simulink model "simulink_3K04"  (R2022a)
settings: Solver=FixedStepAuto  StartTime=0.0  StopTime=10.0  FixedStep=1e-3  RelTol=1e-3  EnableMultiTasking=on
undefined symbols (not defined in the file): D0, D1, D10, D11, D12, D13, D2, D3, D4, D5, D6, D7, D8, D9, PTA0, PTA1, PTA2, PTB23, PTB9, PTC16, PTC17, PTC2, PTC3, PTC4, PTD0, PTD1, PTD2, PTD3
libraries: frdmk64flib x19
settings Model: ExtModeTrigDuration=5  Creator=patri  LastModifiedBy=patri
settings OptimizationCC: EnhancedBackFolding=on  PassReuseOutputArgsAs=Individual arguments  ZeroExternalMemoryAtStartup=off  ZeroInternalMemoryAtStartup=off  MaxStackSize=64  OptimizeBlockOrder=speed  DifferentSizesBufferReuse=on  OptimizationCustomize=off  EfficientTunableParamExpr=on
settings DebuggingCC: ParameterTunabilityLossMsg=error
settings HardwareCC: ProdBitPerPointer=32  ProdBitPerSizeT=32  ProdBitPerPtrDiffT=32  ProdLargestAtomicInteger=Long  ProdLargestAtomicFloat=Double  ProdWordSize=32  ProdHWDeviceType=ARM Compatible->ARM Cortex
settings SFSimCC: MATLABDynamicMemAlloc=off
settings RTWCC: SystemTargetFile=ert.tlc  HardwareBoard=NXP FRDM-K64F  TLCOptions="-aInlineSetEventsForThisBaseRateFcn=TLC_FALSE -aSuppressMultiTaskScheduler=TLC_FALSE  -aRateBasedStepFcn=0"  TemplateMakefile=ert_default_tmf  Toolchain=GNU Tools for ARM Embedded Processors
settings CodeAppCC: ForceParamTrailComments=on  IgnoreCustomStorageClasses=off  OperatorAnnotations=on  SimulinkDataObjDesc=on  SFDataObjDesc=on  InsertBlockDesc=on
settings ERTTargetCC: ExtModeTransport=4  ExtModeMexFile=sendToCommService

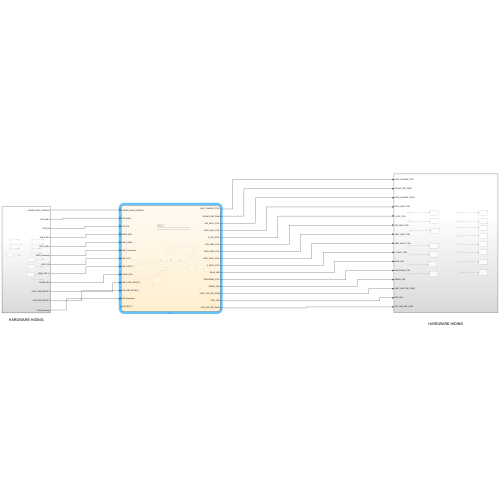
[thumbnail: Simulink's stored preview of the top-level diagram]
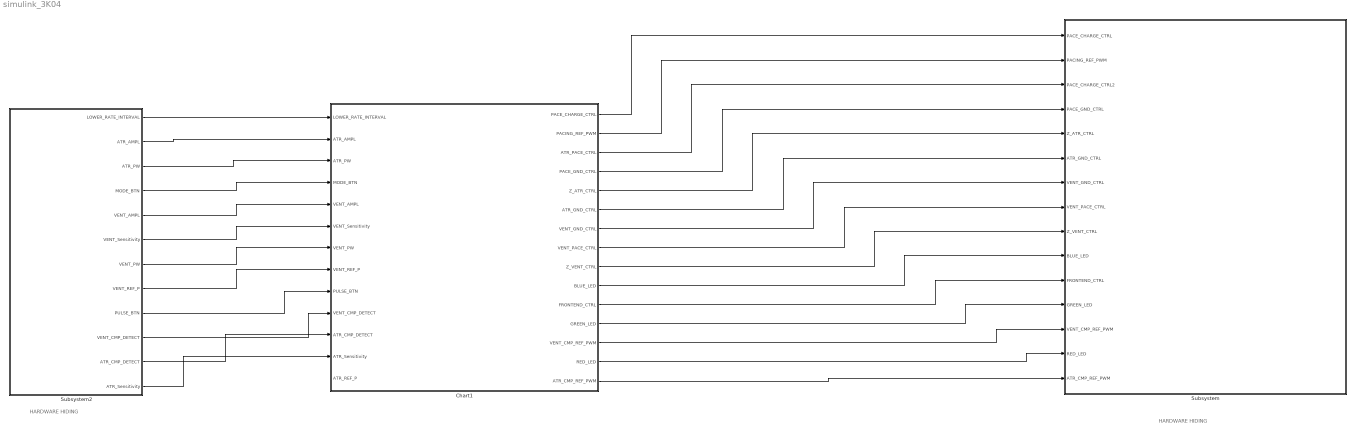
== system simulink_3K04 ==
  note: HARDWARE HIDING
  note: HARDWARE HIDING
  Chart1 : Stateflow chart  TreatAsAtomicUnit=on
  Subsystem : Subsystem
  Subsystem2 : Subsystem
  wires:
  Subsystem2/1(LOWER_RATE_INTERVAL) -> Chart1/1(LOWER_RATE_INTERVAL)
  Chart1/3(ATR_PACE_CTRL) -> Subsystem/3(PACE_CHARGE_CTRL2)
  Chart1/2(PACING_REF_PWM) -> Subsystem/2(PACING_REF_PWM)
  Subsystem2/5(VENT_AMPL) -> Chart1/5(VENT_AMPL)
  Chart1/1(PACE_CHARGE_CTRL) -> Subsystem/1(PACE_CHARGE_CTRL)
  Subsystem2/2(ATR_AMPL) -> Chart1/2(ATR_AMPL)
  Subsystem2/8(VENT_REF_P) -> Chart1/8(VENT_REF_P)
  Chart1/4(PACE_GND_CTRL) -> Subsystem/4(PACE_GND_CTRL)
  Subsystem2/7(VENT_PW) -> Chart1/7(VENT_PW)
  Subsystem2/4(MODE_BTN) -> Chart1/4(MODE_BTN)
  Chart1/7(VENT_GND_CTRL) -> Subsystem/7(VENT_GND_CTRL)
  Chart1/8(VENT_PACE_CTRL) -> Subsystem/8(VENT_PACE_CTRL)
  Chart1/6(ATR_GND_CTRL) -> Subsystem/6(ATR_GND_CTRL)
  Subsystem2/6(VENT_Sensitivity) -> Chart1/6(VENT_Sensitivity)
  Subsystem2/3(ATR_PW) -> Chart1/3(ATR_PW)
  Subsystem2/9(PULSE_BTN) -> Chart1/9(PULSE_BTN)
  Subsystem2/10(VENT_CMP_DETECT) -> Chart1/10(VENT_CMP_DETECT)
  Chart1/11(FRONTEND_CTRL) -> Subsystem/11(FRONTEND_CTRL)
  Chart1/14(RED_LED) -> Subsystem/14(RED_LED)
  Chart1/9(Z_VENT_CTRL) -> Subsystem/9(Z_VENT_CTRL)
  Chart1/12(GREEN_LED) -> Subsystem/12(GREEN_LED)
  Chart1/5(Z_ATR_CTRL) -> Subsystem/5(Z_ATR_CTRL)
  Chart1/13(VENT_CMP_REF_PWM) -> Subsystem/13(VENT_CMP_REF_PWM)
  Chart1/10(BLUE_LED) -> Subsystem/10(BLUE_LED)
  Subsystem2/11(ATR_CMP_DETECT) -> Chart1/11(ATR_CMP_DETECT)
  Chart1/15(ATR_CMP_REF_PWM) -> Subsystem/15(ATR_CMP_REF_PWM)
  Subsystem2/12(ATR_Sensitivity) -> Chart1/12(ATR_Sensitivity)

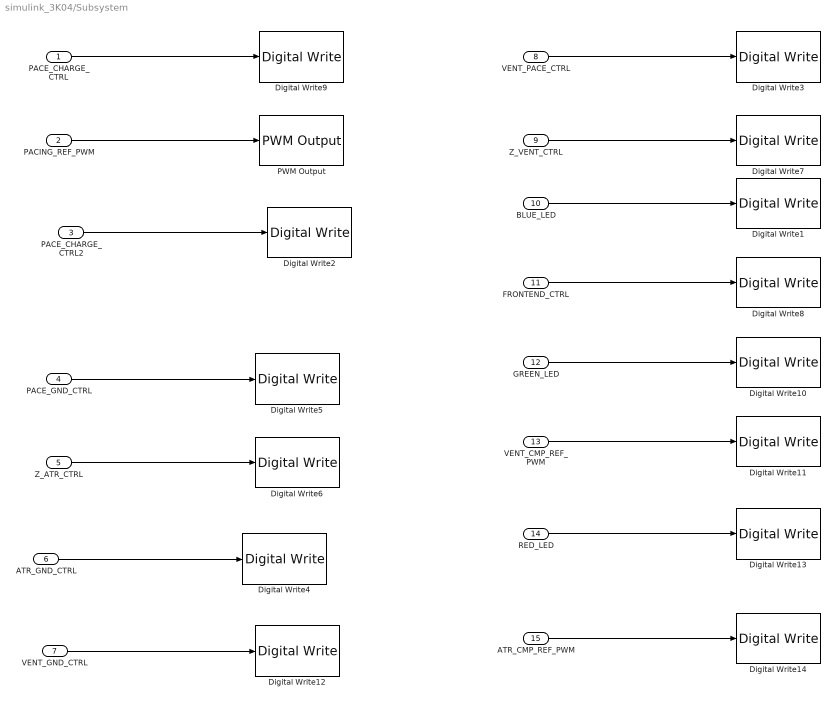
== system simulink_3K04/Subsystem ==
  PACE_CHARGE_CTRL : Inport
  PACING_REF_PWM : Inport  Port=2
  PACE_CHARGE_CTRL2 : Inport  Port=3
  PACE_GND_CTRL : Inport  Port=4
  Z_ATR_CTRL : Inport  Port=5
  ATR_GND_CTRL : Inport  Port=6
  VENT_GND_CTRL : Inport  Port=7
  VENT_PACE_CTRL : Inport  Port=8
  Z_VENT_CTRL : Inport  Port=9
  BLUE_LED : Inport  Port=10
  FRONTEND_CTRL : Inport  Port=11
  GREEN_LED : Inport  Port=12
  VENT_CMP_REF_PWM : Inport  Port=13
  RED_LED : Inport  Port=14
  ATR_CMP_REF_PWM : Inport  Port=15
  Digital Write1 : frdmk64flib/Digital Write  Whichpin=BLUE_LED
  Digital Write10 : frdmk64flib/Digital Write  Whichpin=GREEN_LED
  Digital Write11 : frdmk64flib/Digital Write  Whichpin=PTA1 (D3)
  Digital Write12 : frdmk64flib/Digital Write  Whichpin=PTD3 (D12)
  Digital Write13 : frdmk64flib/Digital Write  Whichpin=RED_LED
  Digital Write14 : frdmk64flib/Digital Write  Whichpin=PTC2 (D6)
  Digital Write2 : frdmk64flib/Digital Write  Whichpin=PTA0 (D8)
  Digital Write3 : frdmk64flib/Digital Write  Whichpin=PTC4 (D9)
  Digital Write4 : frdmk64flib/Digital Write  Whichpin=PTD2 (D11)
  Digital Write5 : frdmk64flib/Digital Write  Whichpin=PTD0 (D10)
  Digital Write6 : frdmk64flib/Digital Write  Whichpin=PTB23 (D4)
  Digital Write7 : frdmk64flib/Digital Write  Whichpin=PTC3 (D7)
  Digital Write8 : frdmk64flib/Digital Write  Whichpin=PTD1 (D13)
  Digital Write9 : frdmk64flib/Digital Write  Whichpin=PTB9 (D2)
  PWM Output : frdmk64flib/PWM Output  Whichpin=PTA2 (D5)  InitialFrequency=2000  InitialDutyCycle=0
  wires:
  PACE_CHARGE_CTRL/1 -> Digital Write9/1
  PACING_REF_PWM/1 -> PWM Output/1
  PACE_CHARGE_CTRL2/1 -> Digital Write2/1
  PACE_GND_CTRL/1 -> Digital Write5/1
  Z_ATR_CTRL/1 -> Digital Write6/1
  ATR_GND_CTRL/1 -> Digital Write4/1
  VENT_GND_CTRL/1 -> Digital Write12/1
  VENT_PACE_CTRL/1 -> Digital Write3/1
  Z_VENT_CTRL/1 -> Digital Write7/1
  BLUE_LED/1 -> Digital Write1/1
  FRONTEND_CTRL/1 -> Digital Write8/1
  GREEN_LED/1 -> Digital Write10/1
  VENT_CMP_REF_PWM/1 -> Digital Write11/1
  RED_LED/1 -> Digital Write13/1
  ATR_CMP_REF_PWM/1 -> Digital Write14/1

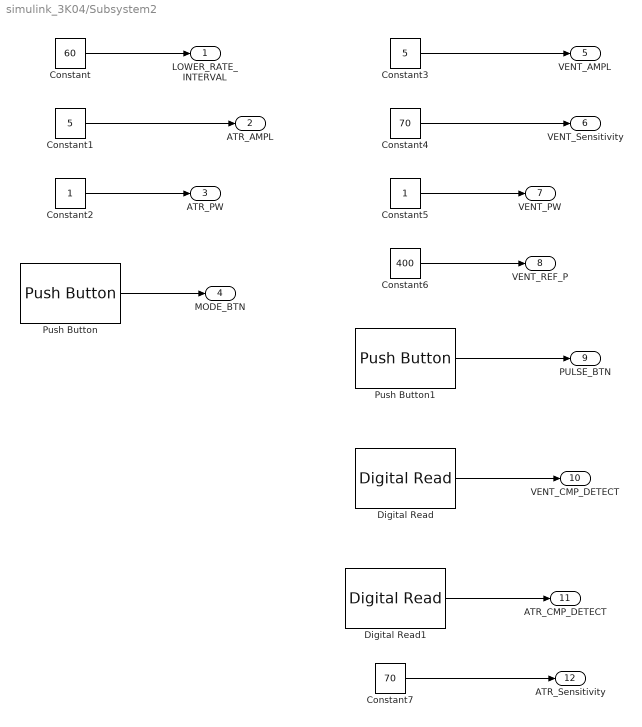
== system simulink_3K04/Subsystem2 ==
  Constant : Constant  Value=60
  Constant1 : Constant  Value=5
  Constant2 : Constant
  Constant3 : Constant  Value=5
  Constant4 : Constant  Value=70
  Constant5 : Constant
  Constant6 : Constant  Value=400
  Constant7 : Constant  Value=70
  Digital Read : frdmk64flib/Digital Read  Whichpin=PTC17 (D1)  SampleTime=-1
  Digital Read1 : frdmk64flib/Digital Read  Whichpin=PTC16 (D0)  SampleTime=-1
  Push Button : frdmk64flib/Push Button  Whichswitch=SW2  SampleTime1=-1
  Push Button1 : frdmk64flib/Push Button  Whichswitch=SW3  SampleTime1=-1
  LOWER_RATE_INTERVAL : Outport
  ATR_AMPL : Outport  Port=2
  ATR_PW : Outport  Port=3
  MODE_BTN : Outport  Port=4
  VENT_AMPL : Outport  Port=5
  VENT_Sensitivity : Outport  Port=6
  VENT_PW : Outport  Port=7
  VENT_REF_P : Outport  Port=8
  PULSE_BTN : Outport  Port=9
  VENT_CMP_DETECT : Outport  Port=10
  ATR_CMP_DETECT : Outport  Port=11
  ATR_Sensitivity : Outport  Port=12
  wires:
  Constant/1 -> LOWER_RATE_INTERVAL/1
  Constant1/1 -> ATR_AMPL/1
  Constant2/1 -> ATR_PW/1
  Push Button/1 -> MODE_BTN/1
  Constant3/1 -> VENT_AMPL/1
  Constant4/1 -> VENT_Sensitivity/1
  Constant5/1 -> VENT_PW/1
  Constant6/1 -> VENT_REF_P/1
  Push Button1/1 -> PULSE_BTN/1
  Digital Read/1 -> VENT_CMP_DETECT/1
  Digital Read1/1 -> ATR_CMP_DETECT/1
  Constant7/1 -> ATR_Sensitivity/1

== stateflow chart simulink_3K04/Chart1 ==
  note: SOLID BLUE LED: AOO
      | SOLID RED LED: VOO
      | BLINKING RED: VVI
      | BLINKING BLUE: AAI
      |
      | STARTS IN AOO, PRESS SW2 BUTTON TO SWITCH MODES, AND SW1 TO RESET BACK TO AOO
      |
      | WHEN IN VVI/AAI, HOLDING SW3 WILL TURN ON GREEN LED AND INHIBIT PACES TO THE HEART
  state PACE_ATR
    entry:
    PACE_CHARGE_CTRL = 0;
    ATR_GND_CTRL = 0;
    ATR_PACE_CTRL = 1;
    BLUE_LED = 1;
  state Charging_C22_AAI
    entry:
    ATR_PACE_CTRL = 0;
    ATR_GND_CTRL = 1;
    PACE_GND_CTRL = 1;
    Z_VENT_CTRL = 0;
    Z_ATR_CTRL = 0;
    FRONTEND_CTRL = 1;
    PACING_REF_PWM = ATR_AMPL*10;
    ATR_CMP_REF_PWM=ATR_Sensitivity;
    VENT_PACE_CTRL = 0;
    VENT_GND_CTRL = 0;
    PACE_CHARGE_CTRL = 1;
    BLUE_LED = 0;
  state REFRACTORY1
    entry:
    BLUE_LED = 0;
    GREEN_LED = 1;
    exit:
    GREEN_LED = 0;
  note: AAI
  state Charging_C22_VOO
    entry:
    VENT_PACE_CTRL = 0;
    VENT_GND_CTRL = 1;
    ATR_PACE_CTRL = 0;
    ATR_GND_CTRL = 0;
    PACE_GND_CTRL = 1;
    Z_VENT_CTRL = 0;
    Z_ATR_CTRL = 0;
    PACE_CHARGE_CTRL = 1;
    RED_LED = 1;
    PACING_REF_PWM = VENT_AMPL*10;
  note: VOO
  note: AOO
  state VENT_Pacing
    entry:
    PACE_CHARGE_CTRL = 0;
    VENT_PACE_CTRL = 1;
    VENT_GND_CTRL = 0;
    RED_LED = 1;
  state MODE
    entry:
    Mode = Mode + 1;
    BLUE_LED = 1;
    RED_LED = 1;
    GREEN_LED = 1;
    exit:
    BLUE_LED = 0;
    RED_LED = 0;
    GREEN_LED = 0;
  state Charging_C22_AOO
    entry:
    VENT_PACE_CTRL = 0;
    VENT_GND_CTRL = 0;
    PACE_GND_CTRL = 1;
    Z_VENT_CTRL = 0;
    Z_ATR_CTRL = 0;
    PACING_REF_PWM = ATR_AMPL*10;
    ATR_PACE_CTRL = 0;
    ATR_GND_CTRL = 1;
    PACE_CHARGE_CTRL = 1;
    BLUE_LED = 1;
  state ATR_Pacing
    entry:
    PACE_CHARGE_CTRL = 0;
    ATR_PACE_CTRL = 1;
    ATR_GND_CTRL = 0;
    BLUE_LED = 1;
  note: VVI
  state PACE_VENT
    entry:
    PACE_CHARGE_CTRL = 0;
    VENT_GND_CTRL = 0;
    VENT_PACE_CTRL = 1;
    RED_LED = 1;
  state Charging_C22_VVI
    entry:
    ATR_PACE_CTRL = 0;
    ATR_GND_CTRL = 0;
    PACE_GND_CTRL = 1;
    Z_VENT_CTRL = 0;
    Z_ATR_CTRL = 0;
    FRONTEND_CTRL = 1;
    PACING_REF_PWM = VENT_AMPL*10;
    VENT_CMP_REF_PWM=VENT_Sensitivity;
    VENT_PACE_CTRL = 0;
    VENT_GND_CTRL = 1;
    PACE_CHARGE_CTRL = 1;
    RED_LED = 0;
  state REFRACTORY
    entry:
    RED_LED = 0;
    GREEN_LED = 1;
    exit:
    GREEN_LED = 0;
  (default) -> Charging_C22_AAI
  Charging_C22_AAI -> PACE_ATR [order 2] : after((60000/LOWER_RATE_INTERVAL)- ATR_PW,msec)
  PACE_ATR -> Charging_C22_AAI : after(ATR_PW,msec)
  REFRACTORY1 -> PACE_ATR [order 2] : after(60000/LOWER_RATE_INTERVAL -  ATR_REF_P + ATR_PW,msec)
  Charging_C22_AAI -> REFRACTORY1 [order 3] : after(ATR_REF_P,msec)[ATR_CMP_DETECT == true || PULSE_BTN == true]
  Charging_C22_AAI -> MODE [order 1] : [MODE_BTN == true]
  MODE -> Charging_C22_AAI [order 1] : [Mode == 4 && MODE_BTN == false]
  REFRACTORY1 -> REFRACTORY1 [order 1] : after(ATR_REF_P,msec)[ATR_CMP_DETECT == true || PULSE_BTN == true]
  Charging_C22_VOO -> MODE [order 2] : [MODE_BTN == true]
  Charging_C22_AOO -> MODE [order 1] : [MODE_BTN == true]
  VENT_Pacing -> Charging_C22_VOO : [after(VENT_PW,msec)]
  MODE -> Charging_C22_VOO [order 4] : [Mode == 2 && MODE_BTN == false]
  Charging_C22_VOO -> VENT_Pacing [order 1] : [after(60000/(LOWER_RATE_INTERVAL)- VENT_PW,msec)]
  ATR_Pacing -> Charging_C22_AOO : after(ATR_PW,msec)
  MODE -> Charging_C22_AOO [order 2] : [Mode == 1 && MODE_BTN == false]
  Charging_C22_VVI -> MODE [order 1] : [MODE_BTN == true]
  MODE -> Charging_C22_VVI [order 3] : [Mode == 3 && MODE_BTN == false]
  Charging_C22_AOO -> ATR_Pacing [order 2] : after((60000/LOWER_RATE_INTERVAL)- ATR_PW,msec)
  PACE_VENT -> Charging_C22_VVI : after(VENT_PW,msec)
  Charging_C22_VVI -> PACE_VENT [order 2] : after((60000/LOWER_RATE_INTERVAL)- VENT_PW,msec)
  REFRACTORY -> PACE_VENT [order 1] : after(60000/LOWER_RATE_INTERVAL - VENT_REF_P + VENT_PW,msec)
  Charging_C22_VVI -> REFRACTORY [order 3] : after(VENT_REF_P,msec)[VENT_CMP_DETECT == true || PULSE_BTN == true]
  REFRACTORY -> REFRACTORY [order 2] : after(VENT_REF_P,msec)[VENT_CMP_DETECT == true || PULSE_BTN == true]
  data: LOWER_RATE_INTERVAL input; PACE_CHARGE_CTRL output; PACING_REF_PWM output; ATR_PACE_CTRL output; PACE_GND_CTRL output; Z_ATR_CTRL output; ATR_GND_CTRL output; VENT_GND_CTRL output; VENT_PACE_CTRL output; Z_VENT_CTRL output; ATR_AMPL input; ATR_PW input; Mode local =0; MODE_BTN input; VENT_AMPL input; BLUE_LED output; VENT_Sensitivity input; FRONTEND_CTRL output; GREEN_LED output; VENT_CMP_REF_PWM output; VENT_PW input; RED_LED output; VENT_REF_P input; PULSE_BTN input; VENT_CMP_DETECT input; ATR_CMP_DETECT input; ATR_CMP_REF_PWM output; ATR_Sensitivity input; ATR_REF_P input
